simulink model "collisionblock"  (R2013a)
settings: Solver=ode45  StartTime=0.0  StopTime=inf  RelTol=1e-3
InitFcn:
  | start_EEVSCube2
  | 
  | %links masses
  | 
  | m=20;%Kg
  | 
  | l=1;%meter
  | 
  | %controls
  | 
  | a=0.3; %singularity positive gain
  | 
  | %Chaser
  | 
  | lb=1;%meter distance 1joint to CM
  | 
  | %Target
  | 
  | mt=750;%kg target mass
  | lt=1;%meter  side lenght
  | It=(1/6)*(lt^2);
  | 
  | %Target Initial Conitions
  | 
  | x_t=2;
  | y_t=3;
  | theta_t=0.7853;
values from neighbouring files (symbols this model uses):
  D = [a b c;d e f;g h i]    [Untitled.m]
undefined symbols (not defined in the file or in its folder): mesh_A, mesh_B
libraries: aerolibanimutils x1
settings Model: Creator=Grompone  LastModifiedBy=Grompone

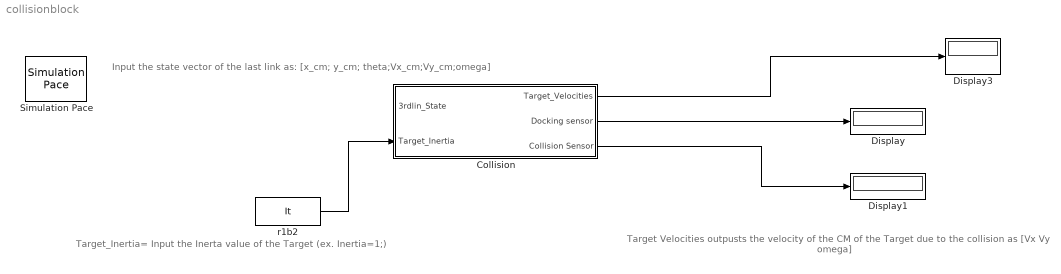
== system collisionblock ==
  note: Target Velocities outpusts the velocity of the CM of the Target due to the collision as [Vx Vy omega]
  note: Input the state vector of the last link as: [x_cm; y_cm; theta;Vx_cm;Vy_cm;omega]
  note: Target_Inertia= Input the Inerta value of the Target (ex. Inertia=1;)
  Collision : Subsystem
  Display : Display
  Display1 : Display
  Display3 : Display
  Simulation Pace : aerolibanimutils/Simulation Pace  SimulationPace=1  SleepMode=MATLAB Thread  OutputPaceError=off  SampleTime=1/30
      settings: AttributesFormatString=%<SimulationPace> sec/sec
  r1b2 : Constant  Value=It
  wires:
  r1b2/1 -> Collision/2(Target_Inertia)
  ? -> Collision/1(3rdlin_State)
  Collision/2(Docking sensor) -> Display/1
  Collision/3(Collision Sensor) -> Display1/1
  Collision/1(Target_Velocities) -> Display3/1

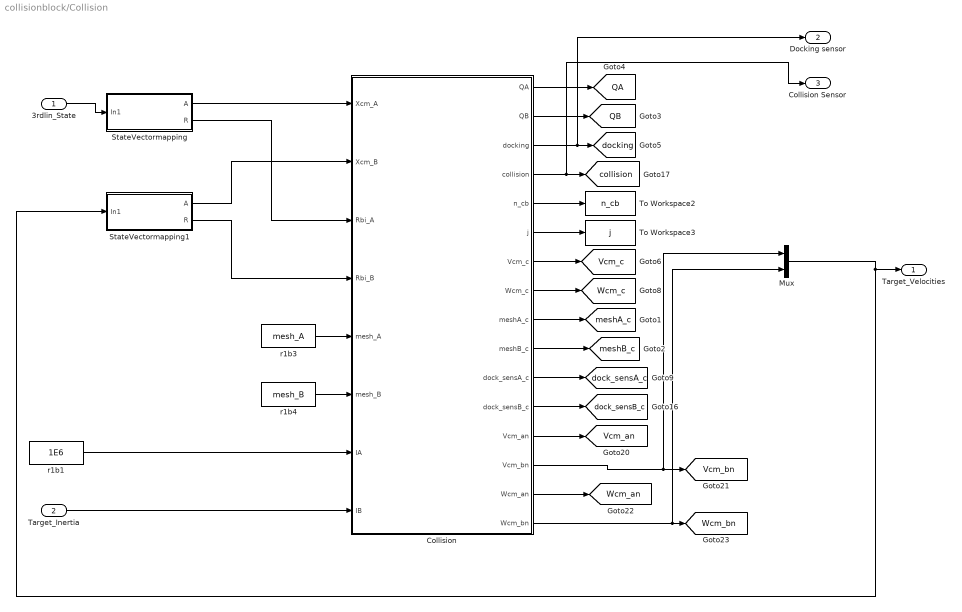
== system collisionblock/Collision ==
  3rdlin_State : Inport
  Target_Inertia : Inport  Port=2
  Collision : Subsystem  mask{mA=1e6, mB=mt, sigma=0.01, sigma_dock=0.1, dotsigma_dock=1, dock_sensA=[0.5 0 0]', dock_sensB=[-0.5 0 0]', epsilon=1}
      mask prompts: mA "Mass of body A [Kg]"; mB "Mass of body B [Kg]"; sigma "Minimum distance for contact [m]"; sigma_dock "Minimum distance for docking (must be greater than contact distance) [m]"; dotsigma_dock "Maximum relative velocity for docking [m/s]"; dock_sensA "Docking sensor position (Body RF) on body A (as [x y z]') [m]"; dock_sensB "Docking sensor position (Body RF) on body B (as [x y z]') [m]"; epsilon "Coefficent of restitution"
      mask help: This block implements collision detection and responce for two rigid bodies of general shapes.
      mask init:
      | ma_mb = [mA; 
      |          mB];
      mask Display:
      | image(imread('collision.jpeg'))
      | color('red');
      | disp('Collision \n Detection and Responce \n v.1.0.9')
      | port_label('input',1,'Xcm_A')
      | port_label('input',2,'Xcm_B')
      | port_label('input',3,'Rbi_A')
      | port_label('input',4,'Rbi_B')
      | port_label('input',5,'mesh_A')
      | port_label('input',6,'mesh_B')
      | port_label('input',7,'IA')
      | port_label('input',8,'IB')
      | 
      | port_label('output',1,'QA')
      | port_label('output',2,'QB')
      | port_label('output',3,'docking')
      | port_label('output',4,'collision')
      | port_label('output',5,'n_cb')
      | port_label('output',6,'j')
      | port_label('output',7,'Vcm_c')
      | port_label('output',8,'Wcm_c')
      | port_label('output',9,'meshA_c')
      | port_label('output',10,'meshB_c')
      | port_label('output',11,'dock_sensA_c')
      | port_label('output',12,'dock_sensB_c')
      | port_label('output',13,'Vcm_an')
      | port_label('output',14,'Vcm_bn')
      | port_label('output',15,'Wcm_an')
      | port_label('output',16,'Wcm_bn')
  Mux : Mux  Inputs=2
  StateVectormapping : Subsystem
  StateVectormapping1 : Subsystem
  To Workspace2 : ToWorkspace  VariableName=n_cb  SampleTime=-1
  To Workspace3 : ToWorkspace  VariableName=j  SampleTime=-1
  r1b1 : Constant  Value=1E6
  r1b3 : Constant  Value=mesh_A
  r1b4 : Constant  Value=mesh_B
  Target_Velocities : Outport
  Docking sensor : Outport  Port=2
  Collision Sensor : Outport  Port=3
  tag scope: QA=global, QB=global, Vcm_an=global, Vcm_bn=global, Vcm_c=global, Wcm_an=global, Wcm_bn=global, Wcm_c=global, collision=global, dock_sensA_c=global, dock_sensB_c=global, docking=global, meshA_c=global, meshB_c=global
  wires:
  Collision/1(QA) -> [QA]
  Collision/2(QB) -> [QB]
  Collision/3(docking) -> Docking sensor/1, [docking]
  Collision/6(j) -> To Workspace3/1
  Collision/4(collision) -> Collision Sensor/1, [collision]
  StateVectormapping/2(R) -> Collision/3(Rbi_A)
  StateVectormapping1/2(R) -> Collision/4(Rbi_B)
  r1b3/1 -> Collision/5(mesh_A)
  r1b4/1 -> Collision/6(mesh_B)
  Collision/5(n_cb) -> To Workspace2/1
  Collision/7(Vcm_c) -> [Vcm_c]
  Collision/8(Wcm_c) -> [Wcm_c]
  Collision/9(meshA_c) -> [meshA_c]
  Collision/10(meshB_c) -> [meshB_c]
  Collision/11(dock_sensA_c) -> [dock_sensA_c]
  Collision/12(dock_sensB_c) -> [dock_sensB_c]
  r1b1/1 -> Collision/7(IA)
  Collision/13(Vcm_an) -> [Vcm_an]
  Collision/15(Wcm_an) -> [Wcm_an]
  Collision/16(Wcm_bn) -> Mux/2, [Wcm_bn]
  3rdlin_State/1 -> StateVectormapping/1(In1)
  StateVectormapping1/1(A) -> Collision/2(Xcm_B)
  Collision/14(Vcm_bn) -> Mux/1, [Vcm_bn]
  Target_Inertia/1 -> Collision/8(IB)
  StateVectormapping/1(A) -> Collision/1(Xcm_A)
  Mux/1 -> StateVectormapping1/1(In1), Target_Velocities/1

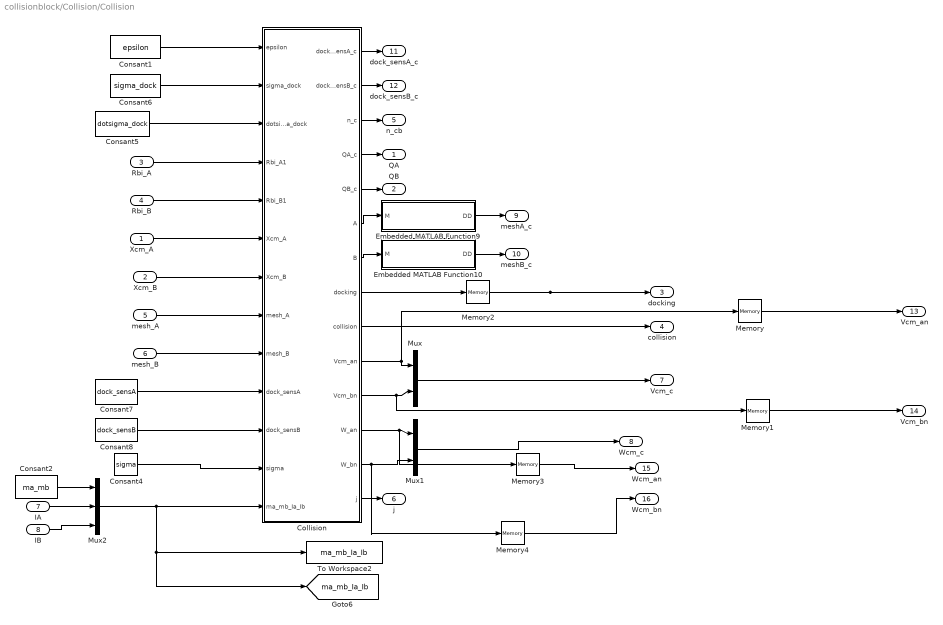
== system collisionblock/Collision/Collision ==
  Xcm_A : Inport
  Xcm_B : Inport  Port=2
  Rbi_A : Inport  Port=3
  Rbi_B : Inport  Port=4
  mesh_A : Inport  Port=5
  mesh_B : Inport  Port=6
  IA : Inport  Port=7
  IB : Inport  Port=8
  Collision : MATLAB Function  TreatAsAtomicUnit=on
  Consant1 : Constant  Value=epsilon
  Consant2 : Constant  Value=ma_mb
  Consant4 : Constant  Value=sigma
  Consant5 : Constant  Value=dotsigma_dock
  Consant6 : Constant  Value=sigma_dock
  Consant7 : Constant  Value=dock_sensA
  Consant8 : Constant  Value=dock_sensB
  Embedded MATLAB Function10 : MATLAB Function  TreatAsAtomicUnit=on
  Embedded MATLAB Function9 : MATLAB Function  TreatAsAtomicUnit=on
  Memory{,1,3..4} (4 alike) : Memory  X0=zeros(3,1)
  Memory2 : Memory
  Mux : Mux  Inputs=2
  Mux1 : Mux  Inputs=2
  Mux2 : Mux  Inputs=3
  To Workspace2 : ToWorkspace  VariableName=ma_mb_Ia_Ib  SampleTime=-1
  QA : Outport
  QB : Outport  Port=2
  docking : Outport  Port=3
  collision : Outport  Port=4
  n_cb : Outport  Port=5
  j : Outport  Port=6
  Vcm_c : Outport  Port=7
  Wcm_c : Outport  Port=8
  meshA_c : Outport  Port=9
  meshB_c : Outport  Port=10
  dock_sensA_c : Outport  Port=11
  dock_sensB_c : Outport  Port=12
  Vcm_an : Outport  Port=13
  Vcm_bn : Outport  Port=14
  Wcm_an : Outport  Port=15
  Wcm_bn : Outport  Port=16
  tag scope: ma_mb_Ia_Ib=global
  wires:
  Embedded MATLAB Function9/1(DD) -> meshA_c/1
  Embedded MATLAB Function10/1(DD) -> meshB_c/1
  Collision/6(A) -> Embedded MATLAB Function9/1(M)
  Collision/7(B) -> Embedded MATLAB Function10/1(M)
  Rbi_B/1 -> Collision/5(Rbi_B1)
  Xcm_A/1 -> Collision/6(Xcm_A)
  mesh_A/1 -> Collision/8(mesh_A)
  mesh_B/1 -> Collision/9(mesh_B)
  Collision/3(n_c) -> n_cb/1
  Collision/8(docking) -> Memory2/1
  Collision/10(Vcm_an) -> Mux/1, Memory/1
  Collision/13(W_bn) -> Mux1/2, Memory4/1
  Collision/14(j) -> j/1
  Collision/9(collision) -> collision/1
  Mux/1 -> Vcm_c/1
  Mux1/1 -> Wcm_c/1
  Collision/4(QA_c) -> QA/1
  Collision/5(QB_c) -> QB/1
  Collision/11(Vcm_bn) -> Memory1/1, Mux/2
  Collision/12(W_an) -> Memory3/1, Mux1/1
  Xcm_B/1 -> Collision/7(Xcm_B)
  Collision/2(dock_sensB_c) -> dock_sensB_c/1
  Collision/1(dock_sensA_c) -> dock_sensA_c/1
  Consant4/1 -> Collision/12(sigma)
  Consant5/1 -> Collision/3(dotsigma_dock)
  Rbi_A/1 -> Collision/4(Rbi_A1)
  Consant6/1 -> Collision/2(sigma_dock)
  Consant7/1 -> Collision/10(dock_sensA)
  Consant8/1 -> Collision/11(dock_sensB)
  Consant1/1 -> Collision/1(epsilon)
  Mux2/1 -> Collision/13(ma_mb_Ia_Ib), To Workspace2/1, [ma_mb_Ia_Ib]
  Consant2/1 -> Mux2/1
  IA/1 -> Mux2/2
  IB/1 -> Mux2/3
  Memory/1 -> Vcm_an/1
  Memory1/1 -> Vcm_bn/1
  Memory3/1 -> Wcm_an/1
  Memory4/1 -> Wcm_bn/1
  Memory2/1 -> docking/1

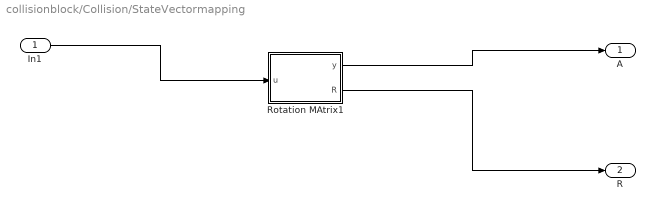
== system collisionblock/Collision/StateVectormapping ==
  In1 : Inport
  Rotation MAtrix1 : MATLAB Function  TreatAsAtomicUnit=on
  A : Outport
  R : Outport  Port=2
  wires:
  Rotation MAtrix1/2(R) -> R/1
  In1/1 -> Rotation MAtrix1/1(u)
  Rotation MAtrix1/1(y) -> A/1

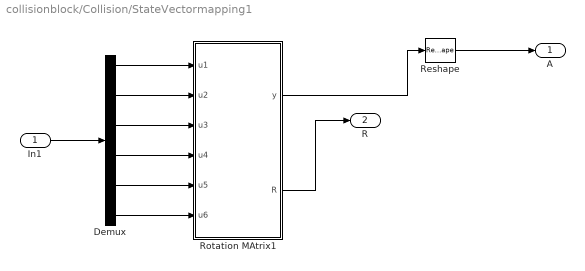
== system collisionblock/Collision/StateVectormapping1 ==
  In1 : Inport
  Demux : Demux  Outputs=6
  Reshape : Reshape  OutputDimensionality=Column vector (2-D)
  Rotation MAtrix1 : MATLAB Function  TreatAsAtomicUnit=on
  A : Outport  PortDimensions=[9,1]
  R : Outport  Port=2
  wires:
  Demux/1 -> Rotation MAtrix1/1(u1)
  Demux/2 -> Rotation MAtrix1/2(u2)
  Demux/3 -> Rotation MAtrix1/3(u3)
  Demux/6 -> Rotation MAtrix1/6(u6)
  Demux/4 -> Rotation MAtrix1/4(u4)
  Demux/5 -> Rotation MAtrix1/5(u5)
  In1/1 -> Demux/1
  Rotation MAtrix1/2(R) -> R/1
  Rotation MAtrix1/1(y) -> Reshape/1
  Reshape/1 -> A/1

== matlab function collisionblock/Collision/Collision/Collision ==
  data: epsilon input; dock_sensA_c output; dock_sensB_c output; n_c output; QA_c output; QB_c output; sigma_dock input; dotsigma_dock input; Rbi_A1 input; Rbi_B1 input; A output; B output; Xcm_A input; Xcm_B input; mesh_A input; mesh_B input; dock_sensA input; dock_sensB input; sigma input; docking output; ma_mb_Ia_Ib input; collision output; Vcm_an output; Vcm_bn output; W_an output; W_bn output; j output
function [dock_sensA_c,dock_sensB_c,n_c,QA_c,QB_c,A,B,docking,collision,Vcm_an,Vcm_bn,W_an,W_bn,j] = fcn(epsilon,sigma_dock,dotsigma_dock,Rbi_A1,Rbi_B1,Xcm_A,Xcm_B,mesh_A,mesh_B,dock_sensA,dock_sensB,sigma,ma_mb_Ia_Ib)

[dock_sensA_c,dock_sensB_c,n_c,QA_c,QB_c,A,B,docking,collision,Vcm_an,Vcm_bn,W_an,W_bn,j] = collision_function(epsilon,sigma_dock,dotsigma_dock,Rbi_A1,Rbi_B1,Xcm_A,Xcm_B,mesh_A,mesh_B,dock_sensA,dock_sensB,sigma,ma_mb_Ia_Ib);

== matlab function collisionblock/Collision/Collision/Embedded MATLAB Function10 ==
  data: M input; DD output
function DD=fcn(M)

[m,n] = size(M);
a = zeros(n*m,1);
MM=zeros(n*m,1);
i=1;
for mm=0:m:n*m-1
for j=1:1:m
    a(j+mm,1)=M(j,i); 
end
i=i+1;
end
DD=a;

== matlab function collisionblock/Collision/Collision/Embedded MATLAB Function9 ==
  data: M input; DD output
function DD=fcn(M)

[m,n] = size(M);
a = zeros(n*m,1);
MM=zeros(n*m,1);
i=1;
for mm=0:m:n*m-1
for j=1:1:m
    a(j+mm,1)=M(j,i); 
end
i=i+1;
end
DD=a;

== matlab function collisionblock/Collision/StateVectormapping/Rotation MAtrix1 ==
  data: u input; y output; R output
function [y,R] = fcn(u)
%#codegen

y=[u(1);u(2); 0; u(4); u(5); 0; 0; 0; u(6)];



R = [cos(u(3)) -sin(u(3));
    sin(u(3)) cos(u(3))];

end

== matlab function collisionblock/Collision/StateVectormapping1/Rotation MAtrix1 ==
  data: u1 input; y output; R output; u2 input; u3 input; u4 input; u5 input; u6 input
function [y,R] = fcn(u1,u2,u3,u4,u5,u6)
%#codegen

% y=[u(1);u(2); 0; u(4); u(5); 0; 0; u(6)];

y=[u1;u2;0;u4;u5;0;0;0;u6];
theta=u3;

R = [cos(theta) -sin(theta);
    sin(theta) cos(theta)];

end
